simulink model "F16"  (R2023b)
settings: Solver=VariableStepAuto  StartTime=0.0  StopTime=120  RelTol=1e-3
libraries: aerolibasang x2, simulink_extras x2, aerolibanim x1
(part 1 of 3)
settings Model: Creator=TADTAWAN  LastModifiedBy=TADTAWAN

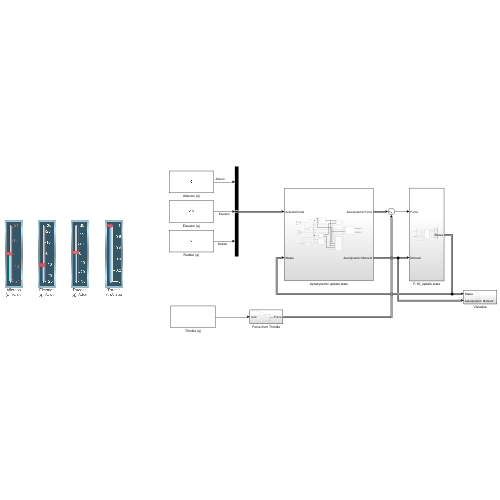
[thumbnail: Simulink's stored preview of the top-level diagram]
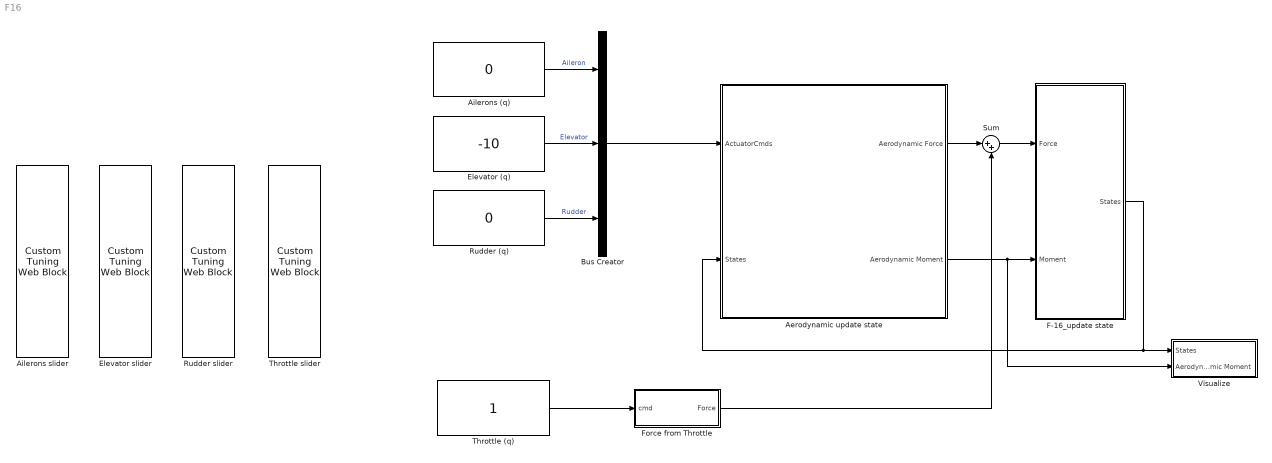
== system F16 ==
  Aerodynamic update state : Subsystem
  Ailerons (q) : Constant  Value=0
  Ailerons slider : CustomTuningWebBlock  LabelPosition=Bottom  ShowInitialText=on  Configuration="{\"components\":[{\"name\":\"LinearScaleComponent\",\"settings\":{\"bounds\":{\"max\":21.5,\"min\":-21.5,\"tickInterval\":\"auto\"},\"internalTickHeightScaleFactor\":0.5,\"labelColor\":[181,82,43],\"labelFont\":{\"font\":\"Arial\",\"fontSize\":12},\"labelOffset\":0.05,\"labelTransparency\":1,\"needleImage\":{\"size\":[596,842],\"src\":\"data:image\\/svg+xml;base64,PD94bWwgdmVyc2lvbj0iMS4wIiBlbmNvZGluZz0idXRmLTgiPz4NCjwhLS0gR2VuZXJhdG9yOiBBZG9iZSBJbGx1c3RyYXRvciAyNS4wLjAsIFNWRyBFeHBvcnQgUGx1Zy1JbiAuIFNWRyBWZXJzaW9uOiA2LjAwIEJ1aWxkIDApICAtLT4NCjxzdmcgdmVyc2lvbj0iMS4xIg0KCSBpZD0ic3ZnOCIgeG1sbnM6Y2M9Imh0dHA6Ly9jcmVhdGl2ZWNvbW1vbnMub3JnL25zIyIgeG1sbnM6ZGM9Imh0dHA6Ly9wdXJsLm9yZy9kYy9lbGVtZW50cy8xLjEvIiB4bWxuczppbmtzY2FwZT0iaHR0cDovL3d3dy5pbmtzY2FwZS5vcmcvbmFtZXNw ...(+2420 chars)\",\"srcOrientation\":\"horizontal\"},\"needleOffset\":[0.0642123287671233,-0.8044596912521441],\"needleSize\":{\"height\":0.07668067226890757,\"width\":0.4337797619047619},\"position\":[0.03623949579831933,0.2829861111111111,0.6088789682539683,0.9196428571428571],\"referencePoint\":\"auto\",\"scaleColors\":[],\"scaleColorsSize\":0.2,\"scaleDirection\":\"BT\",\"showLabels\":1,\"showMinorTicks\":0,\"showSpanLine\":1,\"showTicks\":1,\"tickColor\":[150,61,168],\"tickTransparency\":1,\"valueBarColor\":[15,255,255],\"valueBarOffset\":-0.27,\"valueBarSize\":0.1,\"valueBarTransparency\":1}},{\"name\":\"BackgroundImageComponent\",\"settings\":{\"image\":{\"size\":[380,101],\"src\":\"data:image\\/svg+xml;base64,PHN2ZyB4bWxucz0iaHR0cDovL3d3dy53My5vcmcvMjAwMC9zdmciIHhtbG5zOnhsaW5rPSJodHRwOi8vd3d3LnczLm9yZy8xOTk5L3hsaW5rIiB2aWV3Qm94PSIwIDAgMzgwIDEwMSI+PGRlZnM+PHN0eWxlPi5jbHMtMXtmaWxsOiMwMDJiNDI7fS5jbHMtMntmaWxsOiM0MjcwODI7fS5jbHMtM3tmaWxsOnVybCgjcmFkaWFsLWdyYWRpZW50KTt9LmNscy00e2ZpbGw6I2M4YzhjODtzdHJva2U6IzAwMDt9PC9zdHlsZT48cmFkaWFsR3JhZGllbnQgaWQ9InJhZGlhbC1ncmFkaWVudCIgY3g9IjE5MCIgY3k9IjUwLjUiIHI9IjI2OS4yMSIgZ3JhZGllbnRVbml0cz0idXNlclNwYWNlT25Vc2UiPjxzdG9wIG9mZnNldD0iMC4wMSIgc3RvcC1jb2xvcj0iIzNlNGY1OCIvPjxzdG9wIG9mZnNldD0iMC4wNiIgc3RvcC1jb2xvcj0iIzQ0NTc2MSIvPjxzdG9wIG9mZnNldD0iMC4xNSIgc3RvcC1jb2xvcj0iIzU1NmE3NiIvPjxzdG9wIG9mZnNldD0iMC4yNSIgc3RvcC1jb2xvcj0iIzZkODg5NSIvPjxzdG9wIG9mZnNldD0iMC4zOCIgc3RvcC1jb2xvcj0iIzhmYjJjMyIvPjxzdG9wIG9mZnNldD0iMC41MiIgc3RvcC1jb2xvcj0iI2I2ZTRmYSIvPjxzdG9wIG9mZnNldD0iMSIgc3RvcC1jb2xvcj0iIzE1NDY1NyIvPjwvcmFkaWFsR3JhZGllbnQ+PC9kZWZzPjxnIGlkPSJmcmFtZSI+PGcgaWQ9IkxheWVyXzIiIGRhdGEtbmFtZT0iTGF5ZXIgMiI+PGcgaWQ9IkxheWVyXzEtMiIgZGF0YS1uYW1lPSJMYXllciAxLTIiPjxyZWN0IGlkPSJyZWN0MTAzNiIgY2xhc3M9ImNscy0xIiB4PSIxMSIgeT0iMTEiIHdpZHRoPSIzNTgiIGhlaWdodD0iNzkiLz48cGF0aCBpZD0icGF0aDEwMzgiIGNsYXNzPSJjbHMtMiIgZD0iTTgsOFY5M0gzNzJWOFpNMzY5LDkwSDExVjExSDM2OVoiLz48cGF0aCBpZD0icGF0aDEwNDAiIGNsYXNzPSJjbHMtMyIgZD0iTTAsMFYxMDFIMzgwVjBaTTM3Miw5M0g4VjhIMzcyWiIvPjwvZz48L2c+PC9nPjxnIGlkPSJ0cmFjayI+PHBhdGggaWQ9InJlY3QxNjExIiBjbGFzcz0iY2xzLTQiIGQ9Ik0zMy4zNywyNi41OUgzNDYuNjNjNCwwLDcuMjUsMi42LDcuMjUsNS44MWgwYzAsMy4yMS0zLjI1LDUuODItNy4yNSw1LjgySDMzLjM3Yy00LDAtNy4yNS0yLjYxLTcuMjUtNS44MmgwQzI2LjEyLDI5LjE5LDI5LjM3LDI2LjU5LDMzLjM3LDI2LjU5WiIvPjwvZz48L3N2Zz4=\",\"srcOrientation\":\"horizontal\"},\"position\":[0,0,1,1],\"scaleMode\":\"0\"}},{\"name\":\"ForegroundImageComponent\",\"settings\":{\"image\":{\"size\":[0,0],\"src\":\"default\",\"srcOrientation\":[]},\"isForeground\":1,\"position\":[0,0,1,1],\"scaleMode\":\"0\"}}],\"settings\":{\"BindingType\":\"param\",\"aspectRatio\":3.7777777777777777,\"backgroundColor\":[0,0,0,\"1\"],\"backgroundOffset\":0,\"backgroundOpacity\":1,\"fixedAspectRatio\":\"on\",\"foregroundColor\":[252,252,196],\"orientation\":\"vertical\",\"showBackgroundColor\":false,\"value\":0,\"version\":\"R2023a\"},\"type\":\"LinearGauge\"}"
  Bus Creator : BusCreator  Inputs=3
  Elevator (q) : Constant  Value=-10
  Elevator slider : CustomTuningWebBlock  LabelPosition=Bottom  ShowInitialText=on  Configuration="{\"components\":[{\"name\":\"LinearScaleComponent\",\"settings\":{\"bounds\":{\"max\":25,\"min\":-25,\"tickInterval\":\"auto\"},\"internalTickHeightScaleFactor\":0.5,\"labelColor\":[255,255,200],\"labelFont\":{\"font\":\"Arial\",\"fontSize\":12},\"labelOffset\":0.05,\"labelTransparency\":1,\"needleImage\":{\"size\":[596,842],\"src\":\"data:image\\/svg+xml;base64,PD94bWwgdmVyc2lvbj0iMS4wIiBlbmNvZGluZz0idXRmLTgiPz4NCjwhLS0gR2VuZXJhdG9yOiBBZG9iZSBJbGx1c3RyYXRvciAyNS4wLjAsIFNWRyBFeHBvcnQgUGx1Zy1JbiAuIFNWRyBWZXJzaW9uOiA2LjAwIEJ1aWxkIDApICAtLT4NCjxzdmcgdmVyc2lvbj0iMS4xIg0KCSBpZD0ic3ZnOCIgeG1sbnM6Y2M9Imh0dHA6Ly9jcmVhdGl2ZWNvbW1vbnMub3JnL25zIyIgeG1sbnM6ZGM9Imh0dHA6Ly9wdXJsLm9yZy9kYy9lbGVtZW50cy8xLjEvIiB4bWxuczppbmtzY2FwZT0iaHR0cDovL3d3dy5pbmtzY2FwZS5vcmcvbmFtZXNw ...(+2420 chars)\",\"srcOrientation\":\"horizontal\"},\"needleOffset\":[0.0642123287671233,-0.8044596912521441],\"needleSize\":{\"height\":0.07668067226890757,\"width\":0.4337797619047619},\"position\":[0.03623949579831933,0.2829861111111111,0.6088789682539683,0.9196428571428571],\"referencePoint\":\"auto\",\"scaleColors\":[],\"scaleColorsSize\":0.2,\"scaleDirection\":\"BT\",\"showLabels\":1,\"showMinorTicks\":0,\"showSpanLine\":1,\"showTicks\":1,\"tickColor\":[252,252,197],\"tickTransparency\":1,\"valueBarColor\":[0,114,189],\"valueBarOffset\":-0.27,\"valueBarSize\":0.1,\"valueBarTransparency\":1}},{\"name\":\"BackgroundImageComponent\",\"settings\":{\"image\":{\"size\":[380,101],\"src\":\"data:image\\/svg+xml;base64,PHN2ZyB4bWxucz0iaHR0cDovL3d3dy53My5vcmcvMjAwMC9zdmciIHhtbG5zOnhsaW5rPSJodHRwOi8vd3d3LnczLm9yZy8xOTk5L3hsaW5rIiB2aWV3Qm94PSIwIDAgMzgwIDEwMSI+PGRlZnM+PHN0eWxlPi5jbHMtMXtmaWxsOiMwMDJiNDI7fS5jbHMtMntmaWxsOiM0MjcwODI7fS5jbHMtM3tmaWxsOnVybCgjcmFkaWFsLWdyYWRpZW50KTt9LmNscy00e2ZpbGw6I2M4YzhjODtzdHJva2U6IzAwMDt9PC9zdHlsZT48cmFkaWFsR3JhZGllbnQgaWQ9InJhZGlhbC1ncmFkaWVudCIgY3g9IjE5MCIgY3k9IjUwLjUiIHI9IjI2OS4yMSIgZ3JhZGllbnRVbml0cz0idXNlclNwYWNlT25Vc2UiPjxzdG9wIG9mZnNldD0iMC4wMSIgc3RvcC1jb2xvcj0iIzNlNGY1OCIvPjxzdG9wIG9mZnNldD0iMC4wNiIgc3RvcC1jb2xvcj0iIzQ0NTc2MSIvPjxzdG9wIG9mZnNldD0iMC4xNSIgc3RvcC1jb2xvcj0iIzU1NmE3NiIvPjxzdG9wIG9mZnNldD0iMC4yNSIgc3RvcC1jb2xvcj0iIzZkODg5NSIvPjxzdG9wIG9mZnNldD0iMC4zOCIgc3RvcC1jb2xvcj0iIzhmYjJjMyIvPjxzdG9wIG9mZnNldD0iMC41MiIgc3RvcC1jb2xvcj0iI2I2ZTRmYSIvPjxzdG9wIG9mZnNldD0iMSIgc3RvcC1jb2xvcj0iIzE1NDY1NyIvPjwvcmFkaWFsR3JhZGllbnQ+PC9kZWZzPjxnIGlkPSJmcmFtZSI+PGcgaWQ9IkxheWVyXzIiIGRhdGEtbmFtZT0iTGF5ZXIgMiI+PGcgaWQ9IkxheWVyXzEtMiIgZGF0YS1uYW1lPSJMYXllciAxLTIiPjxyZWN0IGlkPSJyZWN0MTAzNiIgY2xhc3M9ImNscy0xIiB4PSIxMSIgeT0iMTEiIHdpZHRoPSIzNTgiIGhlaWdodD0iNzkiLz48cGF0aCBpZD0icGF0aDEwMzgiIGNsYXNzPSJjbHMtMiIgZD0iTTgsOFY5M0gzNzJWOFpNMzY5LDkwSDExVjExSDM2OVoiLz48cGF0aCBpZD0icGF0aDEwNDAiIGNsYXNzPSJjbHMtMyIgZD0iTTAsMFYxMDFIMzgwVjBaTTM3Miw5M0g4VjhIMzcyWiIvPjwvZz48L2c+PC9nPjxnIGlkPSJ0cmFjayI+PHBhdGggaWQ9InJlY3QxNjExIiBjbGFzcz0iY2xzLTQiIGQ9Ik0zMy4zNywyNi41OUgzNDYuNjNjNCwwLDcuMjUsMi42LDcuMjUsNS44MWgwYzAsMy4yMS0zLjI1LDUuODItNy4yNSw1LjgySDMzLjM3Yy00LDAtNy4yNS0yLjYxLTcuMjUtNS44MmgwQzI2LjEyLDI5LjE5LDI5LjM3LDI2LjU5LDMzLjM3LDI2LjU5WiIvPjwvZz48L3N2Zz4=\",\"srcOrientation\":\"horizontal\"},\"position\":[0,0,1,1],\"scaleMode\":\"0\"}},{\"name\":\"ForegroundImageComponent\",\"settings\":{\"image\":{\"size\":[0,0],\"src\":\"default\",\"srcOrientation\":[]},\"isForeground\":1,\"position\":[0,0,1,1],\"scaleMode\":\"0\"}}],\"settings\":{\"BindingType\":\"param\",\"aspectRatio\":3.7777777777777777,\"backgroundColor\":[0,0,0,\"1\"],\"backgroundOffset\":0,\"backgroundOpacity\":1,\"fixedAspectRatio\":\"on\",\"foregroundColor\":[252,252,196],\"orientation\":\"vertical\",\"showBackgroundColor\":false,\"value\":0,\"version\":\"R2023a\"},\"type\":\"LinearGauge\"}"
  F-16_update state : Subsystem
  Force from Throttle : Subsystem
  Rudder (q) : Constant  Value=0
  Rudder slider : CustomTuningWebBlock  LabelPosition=Bottom  ShowInitialText=on  Configuration="{\"components\":[{\"name\":\"LinearScaleComponent\",\"settings\":{\"bounds\":{\"max\":30,\"min\":-30,\"tickInterval\":\"auto\"},\"internalTickHeightScaleFactor\":0.5,\"labelColor\":[255,255,200],\"labelFont\":{\"font\":\"Arial\",\"fontSize\":12},\"labelOffset\":0.05,\"labelTransparency\":1,\"needleImage\":{\"size\":[596,842],\"src\":\"data:image\\/svg+xml;base64,PD94bWwgdmVyc2lvbj0iMS4wIiBlbmNvZGluZz0idXRmLTgiPz4NCjwhLS0gR2VuZXJhdG9yOiBBZG9iZSBJbGx1c3RyYXRvciAyNS4wLjAsIFNWRyBFeHBvcnQgUGx1Zy1JbiAuIFNWRyBWZXJzaW9uOiA2LjAwIEJ1aWxkIDApICAtLT4NCjxzdmcgdmVyc2lvbj0iMS4xIg0KCSBpZD0ic3ZnOCIgeG1sbnM6Y2M9Imh0dHA6Ly9jcmVhdGl2ZWNvbW1vbnMub3JnL25zIyIgeG1sbnM6ZGM9Imh0dHA6Ly9wdXJsLm9yZy9kYy9lbGVtZW50cy8xLjEvIiB4bWxuczppbmtzY2FwZT0iaHR0cDovL3d3dy5pbmtzY2FwZS5vcmcvbmFtZXNw ...(+2420 chars)\",\"srcOrientation\":\"Right\"},\"needleOffset\":[-0.21513706793802145,-0.7877922077922078],\"needleSize\":{\"height\":0.07666301169590643,\"width\":0.43370508054522927},\"position\":[0.03623949579831933,0.2829861111111111,0.6088789682539683,0.9196428571428571],\"referencePoint\":\"auto\",\"scaleColors\":[],\"scaleColorsSize\":0.2,\"scaleDirection\":\"BT\",\"showLabels\":1,\"showMinorTicks\":0,\"showSpanLine\":1,\"showTicks\":1,\"tickColor\":[252,252,197],\"tickTransparency\":1,\"valueBarColor\":[0,114,189],\"valueBarOffset\":-0.27,\"valueBarSize\":0.1,\"valueBarTransparency\":1}},{\"name\":\"BackgroundImageComponent\",\"settings\":{\"image\":{\"size\":[380,101],\"src\":\"data:image\\/svg+xml;base64,PHN2ZyB4bWxucz0iaHR0cDovL3d3dy53My5vcmcvMjAwMC9zdmciIHhtbG5zOnhsaW5rPSJodHRwOi8vd3d3LnczLm9yZy8xOTk5L3hsaW5rIiB2aWV3Qm94PSIwIDAgMzgwIDEwMSI+PGRlZnM+PHN0eWxlPi5jbHMtMXtmaWxsOiMwMDJiNDI7fS5jbHMtMntmaWxsOiM0MjcwODI7fS5jbHMtM3tmaWxsOnVybCgjcmFkaWFsLWdyYWRpZW50KTt9LmNscy00e2ZpbGw6I2M4YzhjODtzdHJva2U6IzAwMDt9PC9zdHlsZT48cmFkaWFsR3JhZGllbnQgaWQ9InJhZGlhbC1ncmFkaWVudCIgY3g9IjE5MCIgY3k9IjUwLjUiIHI9IjI2OS4yMSIgZ3JhZGllbnRVbml0cz0idXNlclNwYWNlT25Vc2UiPjxzdG9wIG9mZnNldD0iMC4wMSIgc3RvcC1jb2xvcj0iIzNlNGY1OCIvPjxzdG9wIG9mZnNldD0iMC4wNiIgc3RvcC1jb2xvcj0iIzQ0NTc2MSIvPjxzdG9wIG9mZnNldD0iMC4xNSIgc3RvcC1jb2xvcj0iIzU1NmE3NiIvPjxzdG9wIG9mZnNldD0iMC4yNSIgc3RvcC1jb2xvcj0iIzZkODg5NSIvPjxzdG9wIG9mZnNldD0iMC4zOCIgc3RvcC1jb2xvcj0iIzhmYjJjMyIvPjxzdG9wIG9mZnNldD0iMC41MiIgc3RvcC1jb2xvcj0iI2I2ZTRmYSIvPjxzdG9wIG9mZnNldD0iMSIgc3RvcC1jb2xvcj0iIzE1NDY1NyIvPjwvcmFkaWFsR3JhZGllbnQ+PC9kZWZzPjxnIGlkPSJmcmFtZSI+PGcgaWQ9IkxheWVyXzIiIGRhdGEtbmFtZT0iTGF5ZXIgMiI+PGcgaWQ9IkxheWVyXzEtMiIgZGF0YS1uYW1lPSJMYXllciAxLTIiPjxyZWN0IGlkPSJyZWN0MTAzNiIgY2xhc3M9ImNscy0xIiB4PSIxMSIgeT0iMTEiIHdpZHRoPSIzNTgiIGhlaWdodD0iNzkiLz48cGF0aCBpZD0icGF0aDEwMzgiIGNsYXNzPSJjbHMtMiIgZD0iTTgsOFY5M0gzNzJWOFpNMzY5LDkwSDExVjExSDM2OVoiLz48cGF0aCBpZD0icGF0aDEwNDAiIGNsYXNzPSJjbHMtMyIgZD0iTTAsMFYxMDFIMzgwVjBaTTM3Miw5M0g4VjhIMzcyWiIvPjwvZz48L2c+PC9nPjxnIGlkPSJ0cmFjayI+PHBhdGggaWQ9InJlY3QxNjExIiBjbGFzcz0iY2xzLTQiIGQ9Ik0zMy4zNywyNi41OUgzNDYuNjNjNCwwLDcuMjUsMi42LDcuMjUsNS44MWgwYzAsMy4yMS0zLjI1LDUuODItNy4yNSw1LjgySDMzLjM3Yy00LDAtNy4yNS0yLjYxLTcuMjUtNS44MmgwQzI2LjEyLDI5LjE5LDI5LjM3LDI2LjU5LDMzLjM3LDI2LjU5WiIvPjwvZz48L3N2Zz4=\",\"srcOrientation\":\"horizontal\"},\"position\":[0,0,1,1],\"scaleMode\":\"0\"}},{\"name\":\"ForegroundImageComponent\",\"settings\":{\"image\":{\"size\":[0,0],\"src\":\"default\",\"srcOrientation\":[]},\"isForeground\":1,\"position\":[0,0,1,1],\"scaleMode\":\"0\"}}],\"settings\":{\"BindingType\":\"param\",\"aspectRatio\":3.7777777777777777,\"backgroundColor\":[0,0,0,\"1\"],\"backgroundOffset\":0,\"backgroundOpacity\":1,\"fixedAspectRatio\":\"on\",\"foregroundColor\":[252,252,196],\"orientation\":\"vertical\",\"showBackgroundColor\":false,\"value\":0,\"version\":\"R2023a\"},\"type\":\"LinearGauge\"}"
  Sum : Sum  Inputs=|++
  Throttle (q) : Constant
  Throttle slider : CustomTuningWebBlock  LabelPosition=Bottom  ShowInitialText=on  Configuration="{\"components\":[{\"name\":\"LinearScaleComponent\",\"settings\":{\"bounds\":{\"max\":1,\"min\":0,\"tickInterval\":\"auto\"},\"internalTickHeightScaleFactor\":0.5,\"labelColor\":[255,255,200],\"labelFont\":{\"font\":\"Arial\",\"fontSize\":12},\"labelOffset\":0.05,\"labelTransparency\":1,\"needleImage\":{\"size\":[596,842],\"src\":\"data:image\\/svg+xml;base64,PD94bWwgdmVyc2lvbj0iMS4wIiBlbmNvZGluZz0idXRmLTgiPz4NCjwhLS0gR2VuZXJhdG9yOiBBZG9iZSBJbGx1c3RyYXRvciAyNS4wLjAsIFNWRyBFeHBvcnQgUGx1Zy1JbiAuIFNWRyBWZXJzaW9uOiA2LjAwIEJ1aWxkIDApICAtLT4NCjxzdmcgdmVyc2lvbj0iMS4xIg0KCSBpZD0ic3ZnOCIgeG1sbnM6Y2M9Imh0dHA6Ly9jcmVhdGl2ZWNvbW1vbnMub3JnL25zIyIgeG1sbnM6ZGM9Imh0dHA6Ly9wdXJsLm9yZy9kYy9lbGVtZW50cy8xLjEvIiB4bWxuczppbmtzY2FwZT0iaHR0cDovL3d3dy5pbmtzY2FwZS5vcmcvbmFtZXNw ...(+2420 chars)\",\"srcOrientation\":\"horizontal\"},\"needleOffset\":[0.0642123287671233,-0.8044596912521441],\"needleSize\":{\"height\":0.07668067226890757,\"width\":0.4337797619047619},\"position\":[0.03623949579831933,0.2829861111111111,0.6088789682539683,0.9196428571428571],\"referencePoint\":\"auto\",\"scaleColors\":[],\"scaleColorsSize\":0.2,\"scaleDirection\":\"BT\",\"showLabels\":1,\"showMinorTicks\":0,\"showSpanLine\":1,\"showTicks\":1,\"tickColor\":[252,252,197],\"tickTransparency\":1,\"valueBarColor\":[0,114,189],\"valueBarOffset\":-0.27,\"valueBarSize\":0.1,\"valueBarTransparency\":1}},{\"name\":\"BackgroundImageComponent\",\"settings\":{\"image\":{\"size\":[380,101],\"src\":\"data:image\\/svg+xml;base64,PHN2ZyB4bWxucz0iaHR0cDovL3d3dy53My5vcmcvMjAwMC9zdmciIHhtbG5zOnhsaW5rPSJodHRwOi8vd3d3LnczLm9yZy8xOTk5L3hsaW5rIiB2aWV3Qm94PSIwIDAgMzgwIDEwMSI+PGRlZnM+PHN0eWxlPi5jbHMtMXtmaWxsOiMwMDJiNDI7fS5jbHMtMntmaWxsOiM0MjcwODI7fS5jbHMtM3tmaWxsOnVybCgjcmFkaWFsLWdyYWRpZW50KTt9LmNscy00e2ZpbGw6I2M4YzhjODtzdHJva2U6IzAwMDt9PC9zdHlsZT48cmFkaWFsR3JhZGllbnQgaWQ9InJhZGlhbC1ncmFkaWVudCIgY3g9IjE5MCIgY3k9IjUwLjUiIHI9IjI2OS4yMSIgZ3JhZGllbnRVbml0cz0idXNlclNwYWNlT25Vc2UiPjxzdG9wIG9mZnNldD0iMC4wMSIgc3RvcC1jb2xvcj0iIzNlNGY1OCIvPjxzdG9wIG9mZnNldD0iMC4wNiIgc3RvcC1jb2xvcj0iIzQ0NTc2MSIvPjxzdG9wIG9mZnNldD0iMC4xNSIgc3RvcC1jb2xvcj0iIzU1NmE3NiIvPjxzdG9wIG9mZnNldD0iMC4yNSIgc3RvcC1jb2xvcj0iIzZkODg5NSIvPjxzdG9wIG9mZnNldD0iMC4zOCIgc3RvcC1jb2xvcj0iIzhmYjJjMyIvPjxzdG9wIG9mZnNldD0iMC41MiIgc3RvcC1jb2xvcj0iI2I2ZTRmYSIvPjxzdG9wIG9mZnNldD0iMSIgc3RvcC1jb2xvcj0iIzE1NDY1NyIvPjwvcmFkaWFsR3JhZGllbnQ+PC9kZWZzPjxnIGlkPSJmcmFtZSI+PGcgaWQ9IkxheWVyXzIiIGRhdGEtbmFtZT0iTGF5ZXIgMiI+PGcgaWQ9IkxheWVyXzEtMiIgZGF0YS1uYW1lPSJMYXllciAxLTIiPjxyZWN0IGlkPSJyZWN0MTAzNiIgY2xhc3M9ImNscy0xIiB4PSIxMSIgeT0iMTEiIHdpZHRoPSIzNTgiIGhlaWdodD0iNzkiLz48cGF0aCBpZD0icGF0aDEwMzgiIGNsYXNzPSJjbHMtMiIgZD0iTTgsOFY5M0gzNzJWOFpNMzY5LDkwSDExVjExSDM2OVoiLz48cGF0aCBpZD0icGF0aDEwNDAiIGNsYXNzPSJjbHMtMyIgZD0iTTAsMFYxMDFIMzgwVjBaTTM3Miw5M0g4VjhIMzcyWiIvPjwvZz48L2c+PC9nPjxnIGlkPSJ0cmFjayI+PHBhdGggaWQ9InJlY3QxNjExIiBjbGFzcz0iY2xzLTQiIGQ9Ik0zMy4zNywyNi41OUgzNDYuNjNjNCwwLDcuMjUsMi42LDcuMjUsNS44MWgwYzAsMy4yMS0zLjI1LDUuODItNy4yNSw1LjgySDMzLjM3Yy00LDAtNy4yNS0yLjYxLTcuMjUtNS44MmgwQzI2LjEyLDI5LjE5LDI5LjM3LDI2LjU5LDMzLjM3LDI2LjU5WiIvPjwvZz48L3N2Zz4=\",\"srcOrientation\":\"horizontal\"},\"position\":[0,0,1,1],\"scaleMode\":\"0\"}},{\"name\":\"ForegroundImageComponent\",\"settings\":{\"image\":{\"size\":[0,0],\"src\":\"default\",\"srcOrientation\":[]},\"isForeground\":1,\"position\":[0,0,1,1],\"scaleMode\":\"0\"}}],\"settings\":{\"BindingType\":\"param\",\"aspectRatio\":3.7777777777777777,\"backgroundColor\":[0,0,0,\"1\"],\"backgroundOffset\":0,\"backgroundOpacity\":1,\"fixedAspectRatio\":\"on\",\"foregroundColor\":[252,252,196],\"orientation\":\"vertical\",\"showBackgroundColor\":false,\"value\":0,\"version\":\"R2023a\"},\"type\":\"LinearGauge\"}"
  Visualize : Subsystem
  wires:
  Throttle (q)/1 -> Force from Throttle/1(cmd)
  Bus Creator/1 -> Aerodynamic update state/1(ActuatorCmds)
  F-16_update state/1(States) -> Aerodynamic update state/2(States), Visualize/1(States)
  Force from Throttle/1(Force) -> Sum/2
  Sum/1 -> F-16_update state/1(Force)
  Rudder (q)/1 -> Bus Creator/3  "Rudder"
  Aerodynamic update state/1(Aerodynamic Force) -> Sum/1
  Aerodynamic update state/2(Aerodynamic Moment) -> Visualize/2(Aerodynamic Moment), F-16_update state/2(Moment)
  Elevator (q)/1 -> Bus Creator/2  "Elevator"
  Ailerons (q)/1 -> Bus Creator/1  "Aileron"

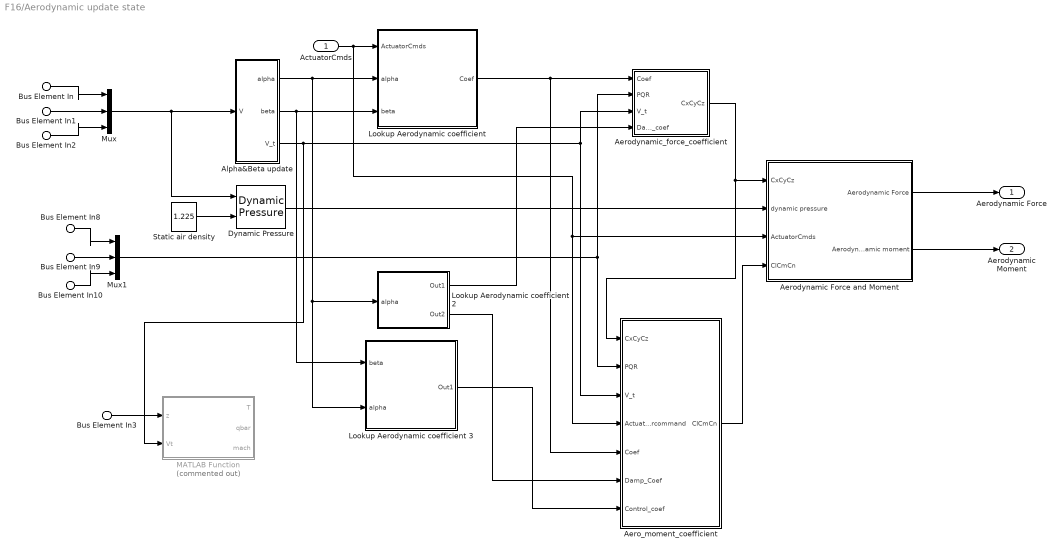
== system F16/Aerodynamic update state ==
  ActuatorCmds : Inport
  Bus Element In : Inport  Port=2  PortName=States  Element=U
  Bus Element In1 : Inport  Port=2  PortName=States  Element=V
  Bus Element In2 : Inport  Port=2  PortName=States  Element=W
  Bus Element In8 : Inport  Port=2  PortName=States  Element=p
  Bus Element In9 : Inport  Port=2  PortName=States  Element=q
  Bus Element In10 : Inport  Port=2  PortName=States  Element=r
  Bus Element In3 : Inport  Port=2  PortName=States  Element=Ze
  Aero_moment_coefficient : Subsystem
  Aerodynamic Force and Moment : Subsystem
  Aerodynamic_force_coefficient : Subsystem
  Alpha&Beta update : Subsystem
  Dynamic Pressure : aerolibasang/Dynamic Pressure
  Lookup Aerodynamic coefficient : Subsystem
  Lookup Aerodynamic coefficient 2 : Subsystem
  Lookup Aerodynamic coefficient 3 : Subsystem
  MATLAB Function : MATLAB Function  Commented=on  TreatAsAtomicUnit=on
  Mux : Mux  Inputs=3
  Mux1 : Mux  Inputs=3
  Static air density : Constant  Value=1.225
  Aerodynamic Force : Outport
  Aerodynamic Moment : Outport  Port=2
  wires:
  Bus Element In1/1 -> Mux/2
  Bus Element In/1 -> Mux/1
  Bus Element In2/1 -> Mux/3
  Mux/1 -> Dynamic Pressure/1, Alpha&Beta update/1(V)
  ActuatorCmds/1 -> Aero_moment_coefficient/4(Actuatorcommand), Aerodynamic Force and Moment/3(ActuatorCmds), Lookup Aerodynamic coefficient/1(ActuatorCmds)
  Static air density/1 -> Dynamic Pressure/2
  Lookup Aerodynamic coefficient/1(Coef) -> Aero_moment_coefficient/5(Coef), Aerodynamic_force_coefficient/1(Coef)
  Aerodynamic Force and Moment/1(Aerodynamic Force) -> Aerodynamic Force/1
  Aerodynamic Force and Moment/2(Aerodynamic moment) -> Aerodynamic Moment/1
  Alpha&Beta update/3(V_t) -> Aerodynamic_force_coefficient/3(V_t), Aero_moment_coefficient/3(V_t), MATLAB Function/2(Vt)
  Mux1/1 -> Aerodynamic_force_coefficient/2(PQR), Aero_moment_coefficient/2(PQR)
  Bus Element In8/1 -> Mux1/1
  Bus Element In9/1 -> Mux1/2
  Bus Element In10/1 -> Mux1/3
  Aerodynamic_force_coefficient/1(CxCyCz) -> Aero_moment_coefficient/1(CxCyCz), Aerodynamic Force and Moment/1(CxCyCz)
  Lookup Aerodynamic coefficient 2/1(Out1) -> Aerodynamic_force_coefficient/4(Damp_coef)
  Lookup Aerodynamic coefficient 2/2(Out2) -> Aero_moment_coefficient/6(Damp_Coef)
  Aero_moment_coefficient/1(ClCmCn) -> Aerodynamic Force and Moment/4(ClCmCn)
  Alpha&Beta update/1(alpha) -> Lookup Aerodynamic coefficient 3/2(alpha), Lookup Aerodynamic coefficient 2/1(alpha), Lookup Aerodynamic coefficient/2(alpha)
  Alpha&Beta update/2(beta) -> Lookup Aerodynamic coefficient 3/1(beta), Lookup Aerodynamic coefficient/3(beta)
  Lookup Aerodynamic coefficient 3/1(Out1) -> Aero_moment_coefficient/7(Control_coef)
  Bus Element In3/1 -> MATLAB Function/1(z)
  Dynamic Pressure/1 -> Aerodynamic Force and Moment/2(dynamic pressure)

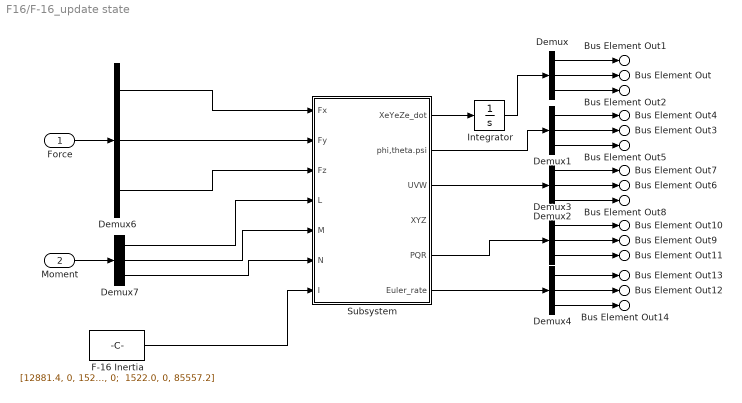
== system F16/F-16_update state ==
  Force : Inport
  Moment : Inport  Port=2
  Demux{,1..4,6..7} (7 alike) : Demux  Outputs=3
  F-16 Inertia : Constant  Value=|
      | [12881.4, 0, 1522.0;
      |  0, 75696.9, 0;
      |  1522.0, 0, 85557.2]
  Integrator : Integrator  InitialCondition=[0;0;-1500]
  Subsystem : Subsystem
  Bus Element Out : Outport  PortName=States  Element=Ye
  Bus Element Out1 : Outport  PortName=States  Element=Xe
  Bus Element Out2 : Outport  PortName=States  Element=Ze
  Bus Element Out3 : Outport  PortName=States  Element=theta
  Bus Element Out4 : Outport  PortName=States  Element=phi
  Bus Element Out5 : Outport  PortName=States  Element=psi
  Bus Element Out6 : Outport  PortName=States  Element=V
  Bus Element Out7 : Outport  PortName=States  Element=U
  Bus Element Out8 : Outport  PortName=States  Element=W
  Bus Element Out9 : Outport  PortName=States  Element=q
  Bus Element Out10 : Outport  PortName=States  Element=p
  Bus Element Out11 : Outport  PortName=States  Element=r
  Bus Element Out12 : Outport  PortName=States  Element=q_dot
  Bus Element Out13 : Outport  PortName=States  Element=p_dot
  Bus Element Out14 : Outport  PortName=States  Element=r_dot
  wires:
  Demux/2 -> Bus Element Out/1
  Demux/1 -> Bus Element Out1/1
  Demux/3 -> Bus Element Out2/1
  Demux1/3 -> Bus Element Out5/1
  Demux1/2 -> Bus Element Out3/1
  Demux1/1 -> Bus Element Out4/1
  Demux2/1 -> Bus Element Out7/1
  Demux2/3 -> Bus Element Out8/1
  Demux2/2 -> Bus Element Out6/1
  Demux3/1 -> Bus Element Out10/1
  Demux3/3 -> Bus Element Out11/1
  Demux3/2 -> Bus Element Out9/1
  Demux4/1 -> Bus Element Out13/1
  Demux4/3 -> Bus Element Out14/1
  Demux4/2 -> Bus Element Out12/1
  Force/1 -> Demux6/1
  Moment/1 -> Demux7/1
  Demux6/1 -> Subsystem/1(Fx)
  Demux6/2 -> Subsystem/2(Fy)
  Demux6/3 -> Subsystem/3(Fz)
  Demux7/1 -> Subsystem/4(L)
  Demux7/2 -> Subsystem/5(M)
  Demux7/3 -> Subsystem/6(N)
  F-16 Inertia/1 -> Subsystem/7(I)
  Subsystem/5(PQR) -> Demux3/1
  Subsystem/2(phi,theta.psi) -> Demux1/1
  Subsystem/3(UVW) -> Demux2/1
  Subsystem/1(XeYeZe_dot) -> Integrator/1
  Integrator/1 -> Demux/1
  Subsystem/6(Euler_rate) -> Demux4/1

== system F16/Force from Throttle ==
  cmd : Inport
  Bus Creator : BusCreator  Inputs=3
  Constant : Constant  Value=0
  Constant1 : Constant  Value=0
  Engine Power : Constant  Value=20500
  F_x : Product
  Force : Outport
  wires:
  Engine Power/1 -> F_x/1
  cmd/1 -> F_x/2
  F_x/1 -> Bus Creator/1  "F_x"
  Constant/1 -> Bus Creator/2  "F_y"
  Constant1/1 -> Bus Creator/3  "F_z"
  Bus Creator/1 -> Force/1

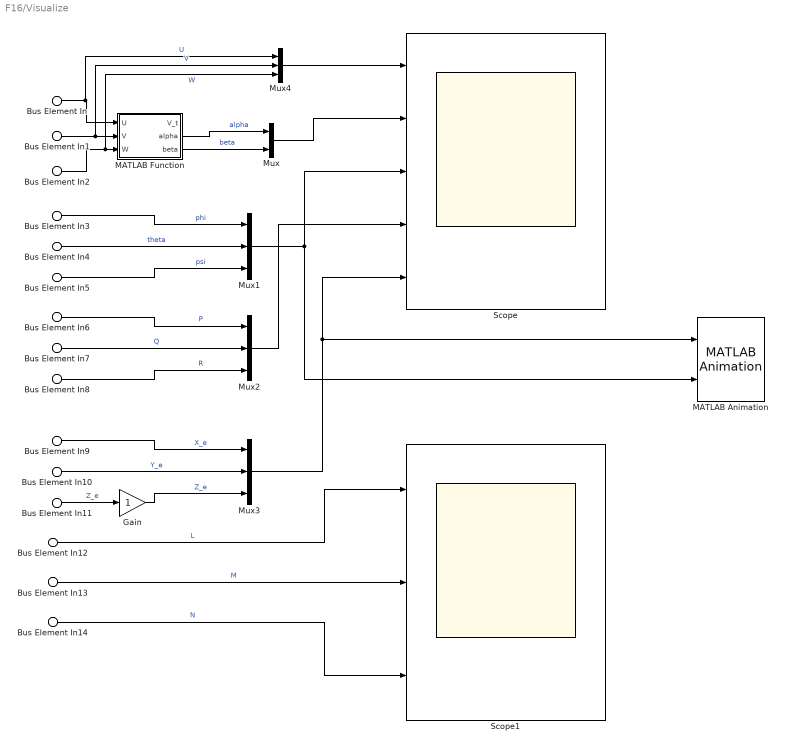
== system F16/Visualize ==
  Bus Element In : Inport  PortName=States  Element=U
  Bus Element In2 : Inport  PortName=States  Element=W
  Bus Element In1 : Inport  PortName=States  Element=V
  Bus Element In3 : Inport  PortName=States  Element=phi
  Bus Element In4 : Inport  PortName=States  Element=theta
  Bus Element In5 : Inport  PortName=States  Element=psi
  Bus Element In6 : Inport  PortName=States  Element=p
  Bus Element In7 : Inport  PortName=States  Element=q
  Bus Element In8 : Inport  PortName=States  Element=r
  Bus Element In9 : Inport  PortName=States  Element=Xe
  Bus Element In10 : Inport  PortName=States  Element=Ye
  Bus Element In11 : Inport  PortName=States  Element=Ze
  Bus Element In12 : Inport  Port=2  PortName=Aerodynamic Moment  Element=L
  Bus Element In13 : Inport  Port=2  PortName=Aerodynamic Moment  Element=M
  Bus Element In14 : Inport  Port=2  PortName=Aerodynamic Moment  Element=N
  Gain : Gain
  MATLAB Animation : aerolibanim/MATLAB Animation  Tag=Matlab Animation 6 DOF  Vehicles=1  Geometries='astredwedge.mat'  BoundingBoxCoordinates=[-50,50,-50,50,-50,50]  CameraOffset=[-150,-50,0]  CameraViewAngle=3  SampleTime=0.2  FigurePosition=[41,251,1536,766]
  MATLAB Function : MATLAB Function  TreatAsAtomicUnit=on
  Mux : Mux  Inputs=2
  Mux{1..4} (4 alike) : Mux  Inputs=3
  Scope : Scope  NumInputPorts=5
  Scope1 : Scope  NumInputPorts=3
  wires:
  Bus Element In/1 -> Mux4/1, MATLAB Function/1(U)  "U"
  Bus Element In1/1 -> MATLAB Function/2(V), Mux4/2  "V"
  Bus Element In2/1 -> Mux4/3, MATLAB Function/3(W)  "W"
  MATLAB Function/2(alpha) -> Mux/1  "alpha"
  MATLAB Function/3(beta) -> Mux/2  "beta"
  Mux/1 -> Scope/2
  Bus Element In4/1 -> Mux1/2  "theta"
  Bus Element In3/1 -> Mux1/1  "phi"
  Bus Element In5/1 -> Mux1/3  "psi"
  Mux1/1 -> MATLAB Animation/2, Scope/3
  Bus Element In8/1 -> Mux2/3  "R"
  Bus Element In7/1 -> Mux2/2  "Q"
  Mux2/1 -> Scope/4
  Bus Element In6/1 -> Mux2/1  "P"
  Bus Element In11/1 -> Gain/1  "Z_e"
  Bus Element In10/1 -> Mux3/2  "Y_e"
  Bus Element In9/1 -> Mux3/1  "X_e"
  Mux3/1 -> Scope/5, MATLAB Animation/1
  Bus Element In13/1 -> Scope1/2  "M"
  Bus Element In12/1 -> Scope1/1  "L"
  Bus Element In14/1 -> Scope1/3  "N"
  Gain/1 -> Mux3/3  "Z_e"
  Mux4/1 -> Scope/1

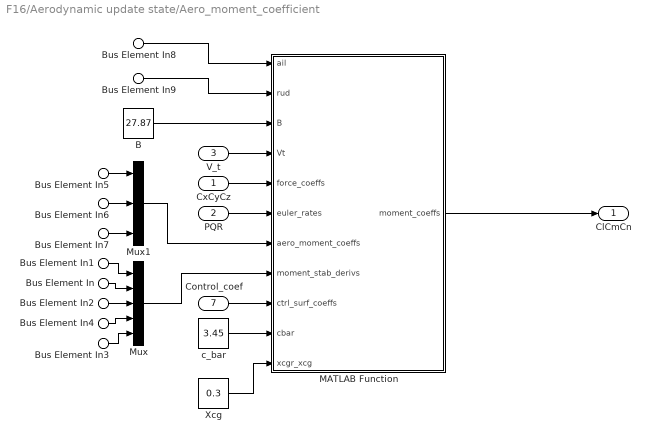
== system F16/Aerodynamic update state/Aero_moment_coefficient ==
  CxCyCz : Inport
  PQR : Inport  Port=2
  V_t : Inport  Port=3
  Bus Element In8 : Inport  Port=4  PortName=Actuatorcommand  Element=Aileron
  Bus Element In9 : Inport  Port=4  PortName=Actuatorcommand  Element=Rudder
  Bus Element In5 : Inport  Port=5  PortName=Coef  Element=c_l
  Bus Element In6 : Inport  Port=5  PortName=Coef  Element=c_m
  Bus Element In7 : Inport  Port=5  PortName=Coef  Element=c_n
  Bus Element In : Inport  Port=6  PortName=Damp_Coef  Element=Clp
  Bus Element In1 : Inport  Port=6  PortName=Damp_Coef  Element=Clr
  Bus Element In2 : Inport  Port=6  PortName=Damp_Coef  Element=Cmp
  Bus Element In3 : Inport  Port=6  PortName=Damp_Coef  Element=Cnp
  Bus Element In4 : Inport  Port=6  PortName=Damp_Coef  Element=Cnr
  Control_coef : Inport  Port=7
  B : Constant  Value=27.87
  MATLAB Function : MATLAB Function  TreatAsAtomicUnit=on
  Mux : Mux  Inputs=5
  Mux1 : Mux  Inputs=3
  Xcg : Constant  Value=0.3
  c_bar : Constant  Value=3.45
  ClCmCn : Outport
  wires:
  MATLAB Function/1(moment_coeffs) -> ClCmCn/1
  Mux/1 -> MATLAB Function/8(moment_stab_derivs)
  Bus Element In2/1 -> Mux/3
  Bus Element In/1 -> Mux/2
  Bus Element In1/1 -> Mux/1
  Bus Element In4/1 -> Mux/4
  Bus Element In3/1 -> Mux/5
  PQR/1 -> MATLAB Function/6(euler_rates)
  Bus Element In7/1 -> Mux1/3
  Bus Element In6/1 -> Mux1/2
  Bus Element In5/1 -> Mux1/1
  Mux1/1 -> MATLAB Function/7(aero_moment_coeffs)
  B/1 -> MATLAB Function/3(B)
  V_t/1 -> MATLAB Function/4(Vt)
  c_bar/1 -> MATLAB Function/10(cbar)
  Xcg/1 -> MATLAB Function/11(xcgr_xcg)
  Bus Element In8/1 -> MATLAB Function/1(ail)
  Bus Element In9/1 -> MATLAB Function/2(rud)
  CxCyCz/1 -> MATLAB Function/5(force_coeffs)
  Control_coef/1 -> MATLAB Function/9(ctrl_surf_coeffs)

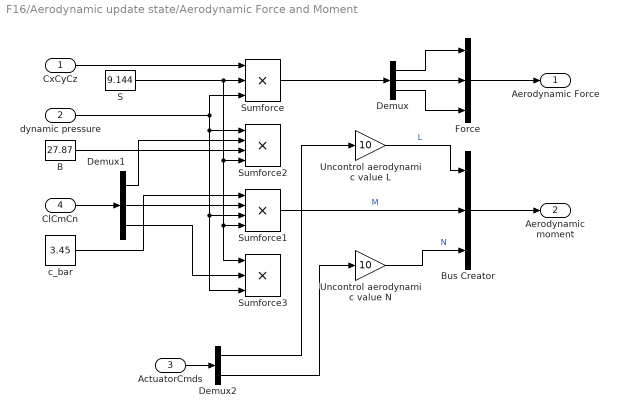
== system F16/Aerodynamic update state/Aerodynamic Force and Moment ==
  CxCyCz : Inport
  dynamic pressure : Inport  Port=2
  ActuatorCmds : Inport  Port=3
  ClCmCn : Inport  Port=4
  B : Constant  Value=27.87
  Bus Creator : BusCreator  Inputs=3
  Demux : Demux  Outputs=3
  Demux1 : Demux  Outputs=3
  Demux2 : Demux  Outputs=3
  Force : BusCreator  Inputs=3
  S : Constant  Value=9.144
  Sumforce : Product  Inputs=3
  Sumforce1 : Product  Inputs=4
  Sumforce2 : Product  Inputs=4
  Sumforce3 : Product  Inputs=3
  Uncontrol aerodynamic value L : Gain  Gain=10
  Uncontrol aerodynamic value N : Gain  Gain=10
  c_bar : Constant  Value=3.45
  Aerodynamic Force : Outport
  Aerodynamic moment : Outport  Port=2
  wires:
  dynamic pressure/1 -> Sumforce3/3, Sumforce1/3, Sumforce2/1, Sumforce/3
  Force/1 -> Aerodynamic Force/1
  CxCyCz/1 -> Sumforce/1
  S/1 -> Sumforce2/4, Sumforce3/1, Sumforce1/4, Sumforce/2
  Sumforce/1 -> Demux/1
  Demux/1 -> Force/1
  Demux/2 -> Force/2
  Demux/3 -> Force/3
  ClCmCn/1 -> Demux1/1
  Demux1/2 -> Sumforce1/2
  Demux1/3 -> Sumforce3/2
  Demux1/1 -> Sumforce2/2
  B/1 -> Sumforce2/3
  c_bar/1 -> Sumforce1/1
  Sumforce1/1 -> Bus Creator/2  "M"
  Bus Creator/1 -> Aerodynamic moment/1
  Uncontrol aerodynamic value L/1 -> Bus Creator/1  "L"
  Uncontrol aerodynamic value N/1 -> Bus Creator/3  "N"
  ActuatorCmds/1 -> Demux2/1
  Demux2/1 -> Uncontrol aerodynamic value L/1
  Demux2/3 -> Uncontrol aerodynamic value N/1

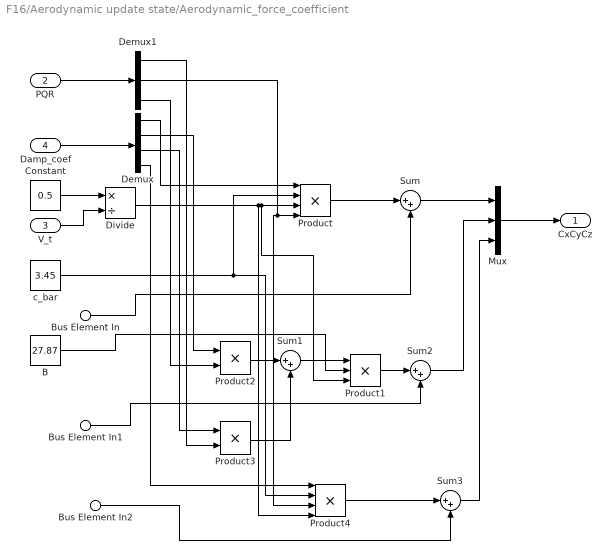
== system F16/Aerodynamic update state/Aerodynamic_force_coefficient ==
  Bus Element In : Inport  PortName=Coef  Element=c_x
  Bus Element In1 : Inport  PortName=Coef  Element=c_y
  Bus Element In2 : Inport  PortName=Coef  Element=c_z
  PQR : Inport  Port=2
  V_t : Inport  Port=3
  Damp_coef : Inport  Port=4
  B : Constant  Value=27.87
  Constant : Constant  Value=0.5
  Demux : Demux
  Demux1 : Demux  Outputs=3
  Divide : Product  Inputs=*/
  Mux : Mux  Inputs=3
  Product : Product  Inputs=4
  Product1 : Product  Inputs=3
  Product2 : Product
  Product3 : Product
  Product4 : Product  Inputs=4
  Sum{,1..3} (4 alike) : Sum  Inputs=|++
  c_bar : Constant  Value=3.45
  CxCyCz : Outport
  wires:
  V_t/1 -> Divide/2
  Constant/1 -> Divide/1
  Damp_coef/1 -> Demux/1
  PQR/1 -> Demux1/1
  Divide/1 -> Product1/3, Product/3, Product4/4
  Bus Element In/1 -> Sum/2
  c_bar/1 -> Product4/2, Product/2
  Demux1/2 -> Product/4, Product4/3
  Product/1 -> Sum/1
  Mux/1 -> CxCyCz/1
  Demux/2 -> Product2/1
  Demux/3 -> Product3/1
  Product2/1 -> Sum1/1
  Product3/1 -> Sum1/2
  Demux/1 -> Product/1
  Sum1/1 -> Product1/1
  B/1 -> Product1/2
  Product1/1 -> Sum2/1
  Bus Element In1/1 -> Sum2/2
  Sum2/1 -> Mux/2
  Sum/1 -> Mux/1
  Demux/4 -> Product4/1
  Product4/1 -> Sum3/1
  Bus Element In2/1 -> Sum3/2
  Sum3/1 -> Mux/3
  Demux1/3 -> Product2/2
  Demux1/1 -> Product3/2

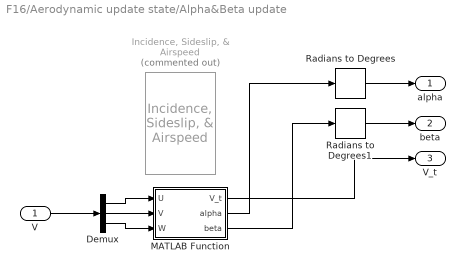
== system F16/Aerodynamic update state/Alpha&Beta update ==
  V : Inport
  Demux : Demux  Outputs=3
  "Incidence, Sideslip, & Airspeed" : aerolibasang/Incidence, Sideslip, & Airspeed  Commented=on
  MATLAB Function : MATLAB Function  TreatAsAtomicUnit=on
  Radians to Degrees : simulink_extras/Transformations/Radians to Degrees
  Radians to Degrees1 : simulink_extras/Transformations/Radians to Degrees
  alpha : Outport
  beta : Outport  Port=2
  V_t : Outport  Port=3
  wires:
  V/1 -> Demux/1
  Demux/1 -> MATLAB Function/1(U)
  Demux/2 -> MATLAB Function/2(V)
  Demux/3 -> MATLAB Function/3(W)
  Radians to Degrees/1 -> alpha/1
  Radians to Degrees1/1 -> beta/1
  MATLAB Function/3(beta) -> Radians to Degrees1/1
  MATLAB Function/2(alpha) -> Radians to Degrees/1
  MATLAB Function/1(V_t) -> V_t/1

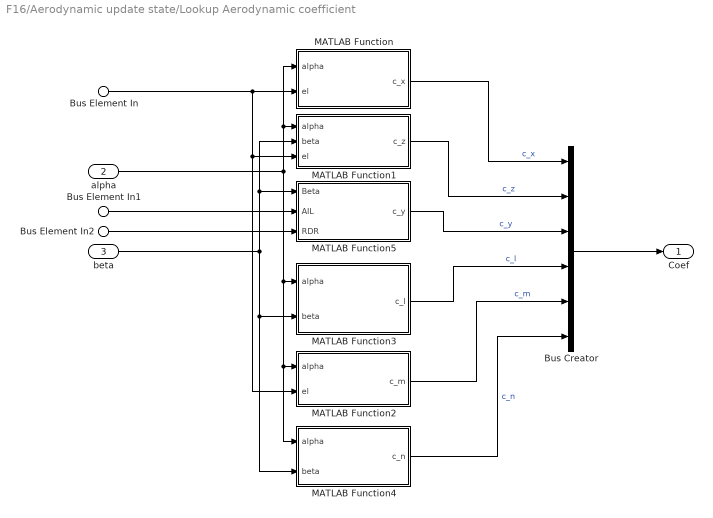
== system F16/Aerodynamic update state/Lookup Aerodynamic coefficient ==
  Bus Element In : Inport  PortName=ActuatorCmds  Element=Elevator
  Bus Element In1 : Inport  PortName=ActuatorCmds  Element=Aileron
  Bus Element In2 : Inport  PortName=ActuatorCmds  Element=Rudder
  alpha : Inport  Port=2
  beta : Inport  Port=3
  Bus Creator : BusCreator  Inputs=6
  MATLAB Function : MATLAB Function  TreatAsAtomicUnit=on
  MATLAB Function1 : MATLAB Function  TreatAsAtomicUnit=on
  MATLAB Function2 : MATLAB Function  TreatAsAtomicUnit=on
  MATLAB Function3 : MATLAB Function  TreatAsAtomicUnit=on
  MATLAB Function4 : MATLAB Function  TreatAsAtomicUnit=on
  MATLAB Function5 : MATLAB Function  TreatAsAtomicUnit=on
  Coef : Outport
  wires:
  Bus Element In1/1 -> MATLAB Function5/2(AIL)
  Bus Element In2/1 -> MATLAB Function5/3(RDR)
  Bus Element In/1 -> MATLAB Function2/2(el), MATLAB Function1/3(el), MATLAB Function/2(el)
  beta/1 -> MATLAB Function4/2(beta), MATLAB Function3/2(beta), MATLAB Function1/2(beta), MATLAB Function5/1(Beta)
  MATLAB Function/1(c_x) -> Bus Creator/1  "c_x"
  MATLAB Function1/1(c_z) -> Bus Creator/2  "c_z"
  alpha/1 -> MATLAB Function4/1(alpha), MATLAB Function2/1(alpha), MATLAB Function3/1(alpha), MATLAB Function/1(alpha), MATLAB Function1/1(alpha)
  Bus Creator/1 -> Coef/1
  MATLAB Function2/1(c_m) -> Bus Creator/5  "c_m"
  MATLAB Function4/1(c_n) -> Bus Creator/6  "c_n"
  MATLAB Function5/1(c_y) -> Bus Creator/3  "c_y"
  MATLAB Function3/1(c_l) -> Bus Creator/4  "c_l"

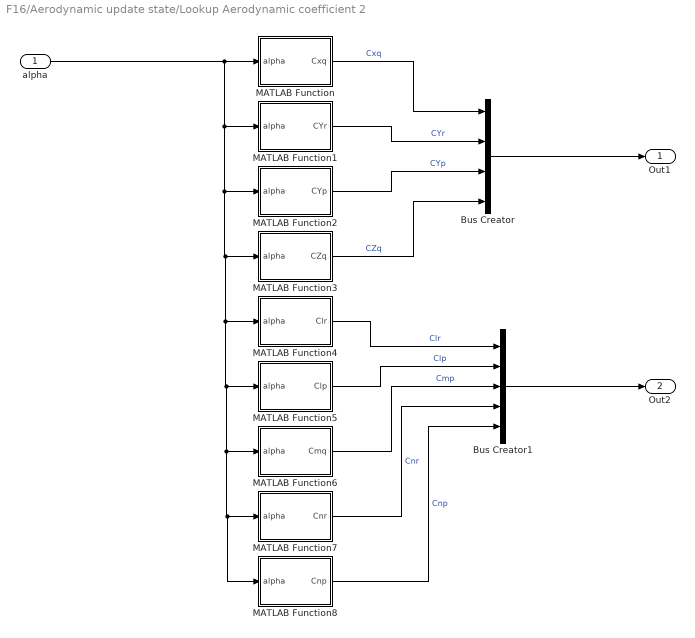
== system F16/Aerodynamic update state/Lookup Aerodynamic coefficient 2 ==
  alpha : Inport
  Bus Creator : BusCreator  Inputs=4
  Bus Creator1 : BusCreator  Inputs=5
  MATLAB Function : MATLAB Function  TreatAsAtomicUnit=on
  MATLAB Function1 : MATLAB Function  TreatAsAtomicUnit=on
  MATLAB Function2 : MATLAB Function  TreatAsAtomicUnit=on
  MATLAB Function3 : MATLAB Function  TreatAsAtomicUnit=on
  MATLAB Function4 : MATLAB Function  TreatAsAtomicUnit=on
  MATLAB Function5 : MATLAB Function  TreatAsAtomicUnit=on
  MATLAB Function6 : MATLAB Function  TreatAsAtomicUnit=on
  MATLAB Function7 : MATLAB Function  TreatAsAtomicUnit=on
  MATLAB Function8 : MATLAB Function  TreatAsAtomicUnit=on
  Out1 : Outport
  Out2 : Outport  Port=2
  wires:
  MATLAB Function4/1(Clr) -> Bus Creator1/1  "Clr"
  MATLAB Function/1(Cxq) -> Bus Creator/1  "Cxq"
  MATLAB Function6/1(Cmq) -> Bus Creator1/3  "Cmp"
  alpha/1 -> MATLAB Function/1(alpha), MATLAB Function8/1(alpha), MATLAB Function7/1(alpha), MATLAB Function6/1(alpha), MATLAB Function5/1(alpha), MATLAB Function4/1(alpha), MATLAB Function3/1(alpha), MATLAB Function2/1(alpha), MATLAB Function1/1(alpha)
  MATLAB Function8/1(Cnp) -> Bus Creator1/5  "Cnp"
  MATLAB Function2/1(CYp) -> Bus Creator/3  "CYp"
  MATLAB Function5/1(Clp) -> Bus Creator1/2  "Clp"
  Bus Creator1/1 -> Out2/1
  MATLAB Function1/1(CYr) -> Bus Creator/2  "CYr"
  MATLAB Function3/1(CZq) -> Bus Creator/4  "CZq"
  Bus Creator/1 -> Out1/1
  MATLAB Function7/1(Cnr) -> Bus Creator1/4  "Cnr"

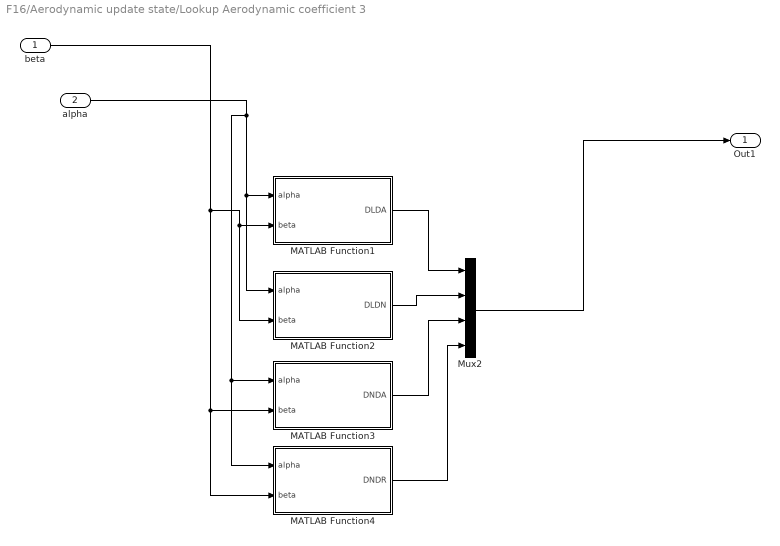
== system F16/Aerodynamic update state/Lookup Aerodynamic coefficient 3 ==
  beta : Inport
  alpha : Inport  Port=2
  MATLAB Function1 : MATLAB Function  TreatAsAtomicUnit=on
  MATLAB Function2 : MATLAB Function  TreatAsAtomicUnit=on
  MATLAB Function3 : MATLAB Function  TreatAsAtomicUnit=on
  MATLAB Function4 : MATLAB Function  TreatAsAtomicUnit=on
  Mux2 : Mux
  Out1 : Outport
  wires:
  MATLAB Function2/1(DLDN) -> Mux2/2
  beta/1 -> MATLAB Function4/2(beta), MATLAB Function3/2(beta), MATLAB Function2/2(beta), MATLAB Function1/2(beta)
  alpha/1 -> MATLAB Function2/1(alpha), MATLAB Function1/1(alpha), MATLAB Function4/1(alpha), MATLAB Function3/1(alpha)
  Mux2/1 -> Out1/1
  MATLAB Function1/1(DLDA) -> Mux2/1
  MATLAB Function3/1(DNDA) -> Mux2/3
  MATLAB Function4/1(DNDR) -> Mux2/4

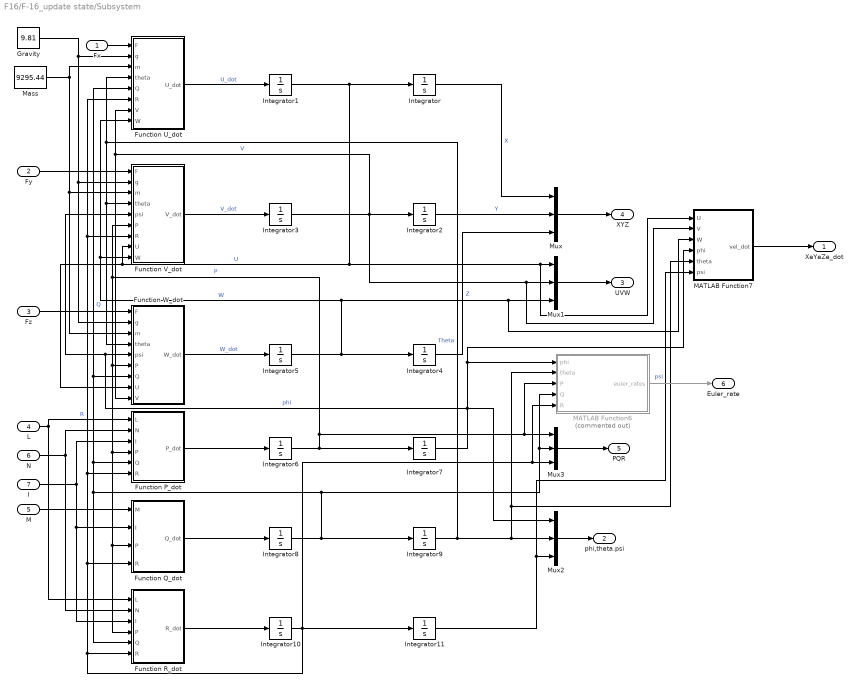
== system F16/F-16_update state/Subsystem ==
  Fx : Inport
  Fy : Inport  Port=2
  Fz : Inport  Port=3
  L : Inport  Port=4
  M : Inport  Port=5
  N : Inport  Port=6
  I : Inport  Port=7
  Function P_dot : MATLAB Function  TreatAsAtomicUnit=on
  Function Q_dot : MATLAB Function  TreatAsAtomicUnit=on
  Function R_dot : MATLAB Function  TreatAsAtomicUnit=on
  Function U_dot : MATLAB Function  TreatAsAtomicUnit=on
  Function V_dot : MATLAB Function  TreatAsAtomicUnit=on
  Function W_dot : MATLAB Function  TreatAsAtomicUnit=on
  Gravity : Constant  Value=9.81
  Integrator{,2,6..8,10..11} (7 alike) : Integrator
  Integrator1 : Integrator  InitialCondition=249.99
  Integrator3 : Integrator  InitialCondition=0.01
  Integrator4 : Integrator  InitialCondition=-1500
  Integrator5 : Integrator  InitialCondition=0.5
  Integrator9 : Integrator  InitialCondition=0.002
  MATLAB Function6 : MATLAB Function  Commented=on  TreatAsAtomicUnit=on
  MATLAB Function7 : MATLAB Function  TreatAsAtomicUnit=on
  Mass : Constant  Value=9295.44
  Mux{,1..3} (4 alike) : Mux  Inputs=3
  XeYeZe_dot : Outport
  phi,theta.psi : Outport  Port=2
  UVW : Outport  Port=3
  XYZ : Outport  Port=4
  PQR : Outport  Port=5
  Euler_rate : Outport  Port=6
  wires:
  Gravity/1 -> Function V_dot/2(g), Function W_dot/2(g), Function U_dot/2(g)
  Integrator3/1 -> Function U_dot/7(V), Function W_dot/9(V), MATLAB Function7/2(V), Mux1/2, Integrator2/1  "V"
  Mass/1 -> Function U_dot/3(m), Function W_dot/3(m), Function V_dot/3(m)
  Integrator6/1 -> Function P_dot/4(P), Function R_dot/4(P), Function Q_dot/3(P), Function W_dot/6(P), Function V_dot/6(P), MATLAB Function6/3(P), Mux3/1, Integrator7/1  "P"
  Integrator5/1 -> MATLAB Function7/3(W), Mux1/3, Function V_dot/9(W), Function U_dot/8(W), Integrator4/1  "W"
  Function P_dot/1(P_dot) -> Integrator6/1
  Integrator10/1 -> MATLAB Function6/5(R), Mux3/3, Function V_dot/7(R), Function U_dot/6(R), Function P_dot/6(R), Function Q_dot/4(R), Function R_dot/6(R), Integrator11/1  "R"
  Function Q_dot/1(Q_dot) -> Integrator8/1
  I/1 -> Function R_dot/3(I), Function Q_dot/2(I), Function P_dot/3(I)
  Integrator1/1 -> Integrator/1, Function W_dot/8(U), Function V_dot/8(U), Mux1/1, MATLAB Function7/1(U)  "U"
  Integrator9/1 -> MATLAB Function6/2(theta), MATLAB Function7/5(theta), Mux2/2, Function U_dot/4(theta), Function V_dot/4(theta), Function W_dot/4(theta)  "Theta"
  N/1 -> Function R_dot/2(N), Function P_dot/2(N)
  Integrator8/1 -> Integrator9/1, Function R_dot/5(Q), Function W_dot/7(Q), Function U_dot/5(Q), Function P_dot/5(Q), MATLAB Function6/4(Q), Mux3/2  "Q"
  Integrator11/1 -> MATLAB Function7/6(psi), Mux2/3  "psi"
  Function R_dot/1(R_dot) -> Integrator10/1
  Fx/1 -> Function U_dot/1(F)
  Function U_dot/1(U_dot) -> Integrator1/1  "U_dot"
  L/1 -> Function R_dot/1(L), Function P_dot/1(L)
  Fy/1 -> Function V_dot/1(F)
  Function W_dot/1(W_dot) -> Integrator5/1  "W_dot"
  Function V_dot/1(V_dot) -> Integrator3/1  "V_dot"
  Integrator2/1 -> Mux/2  "Y"
  Integrator4/1 -> Mux/3  "Z"
  M/1 -> Function Q_dot/1(M)
  Integrator/1 -> Mux/1  "X"
  Integrator7/1 -> Mux2/1, MATLAB Function7/4(phi), MATLAB Function6/1(phi), Function W_dot/5(psi), Function V_dot/5(psi)  "phi"
  Fz/1 -> Function W_dot/1(F)
  Mux/1 -> XYZ/1
  Mux1/1 -> UVW/1
  Mux2/1 -> phi,theta.psi/1
  Mux3/1 -> PQR/1
  MATLAB Function6/1(euler_rates) -> Euler_rate/1
  MATLAB Function7/1(vel_dot) -> XeYeZe_dot/1

== matlab function F16/F-16_update state/Subsystem/Function Q_dot ==
  data: M input; Q_dot output; I input; P input; R input
function Q_dot = fcn(M,I,P,R)
    % Extract inertia components from the 3x3 inertia matrix
    Ixx = I(1,1);
    Iyy = I(2,2);
    Izz = I(3,3);
    Ixz = I(1,3); % Assuming symmetric matrix
    
    % Compute Q_dot
    Q_dot = (M + (Izz - Ixx) * P * R - Ixz * (P^2 - R^2)) / Iyy;

== matlab function F16/F-16_update state/Subsystem/Function R_dot ==
  data: L input; N input; R_dot output; I input; P input; Q input; R input
function R_dot = fcn(L,N,I,P,Q,R)
    % Extract inertia components from the 3x3 inertia matrix
    Ixx = I(1,1);
    Iyy = I(2,2);
    Izz = I(3,3);
    Ixz = I(1,3); % Assuming symmetric matrix
    
    % Compute Gamma
    Gamma = Ixx * Izz - Ixz^2;

    % Compute R_dot
    R_dot = (Ixx * N + Ixz * L - (Ixx * (Ixx - Iyy) + Ixz^2) * P * Q ...
             + Ixz * (Ixx - Iyy + Izz) * Q * R) / Gamma;

    % R_dot = (Ixx * N) / Gamma;

== matlab function F16/F-16_update state/Subsystem/Function U_dot ==
  data: F input; U_dot output; g input; m input; theta input; Q input; R input; V input; W input
function U_dot = fcn(F,g,m,theta,Q,R,V,W)
U_dot = R*V - Q*W - g*sin(theta) + F/m;

== matlab function F16/F-16_update state/Subsystem/Function V_dot ==
  data: F input; V_dot output; g input; m input; theta input; psi input; P input; R input; U input; W input
function V_dot = fcn(F,g,m,theta,psi,P,R,U,W)
    if m == 0
        V_dot = NaN;
        warning('Mass (m) is zero, returning NaN.');
        return;
    end
    % Ensure theta and psi are valid
    if isnan(theta) || isnan(psi)
        V_dot = NaN;
        warning('Theta or Psi is NaN, returning NaN.');
        return;
    end
    V_dot = P*W - R*U + g*cos(theta)*sin(psi) + F/m;
    % V_dot = 0;

== matlab function F16/F-16_update state/Subsystem/Function W_dot ==
  data: F input; W_dot output; g input; m input; theta input; psi input; P input; Q input; U input; V input
function W_dot = fcn(F,g,m,theta,psi,P,Q,U,V)
W_dot = Q*U - P*V + g*cos(theta)*cos(psi) + F/m;

== matlab function F16/F-16_update state/Subsystem/MATLAB Function6 ==
  data: phi input; euler_rates output; theta input; P input; Q input; R input
function euler_rates = fcn(phi, theta, P, Q, R)
if abs(cos(theta)) < 1e-6
    error('Theta is near ±pi/2, causing a singularity.');
end

T = [1, sin(phi)*tan(theta), cos(phi)*tan(theta);
     0, cos(phi), -sin(phi);
     0, sin(phi)/cos(theta), cos(phi)/cos(theta)];

angular_velocity = [P; Q; R];

euler_rates = T * angular_velocity;
end
